simulink model "FOC_ctrl"  (R2025b)
settings: Solver=FixedStepAuto  StartTime=0.0  StopTime=Tstop  FixedStep=p.FastTs  RelTol=1e-3
undefined symbols (not defined in the file): angleDeg, c, Inverter, m, Motor, p, torqueNm, Tstop, we
libraries: simulink x5, fl_lib x4, nesl_utility x3, dspsigops x2, ee_lib x1
(part 1 of 3)
Description:
  | Release 2.0.11
settings Model: Creator=dehc5899  LastModifiedBy=dehc5899
settings SolverCC: AutoInsertRateTranBlk=on

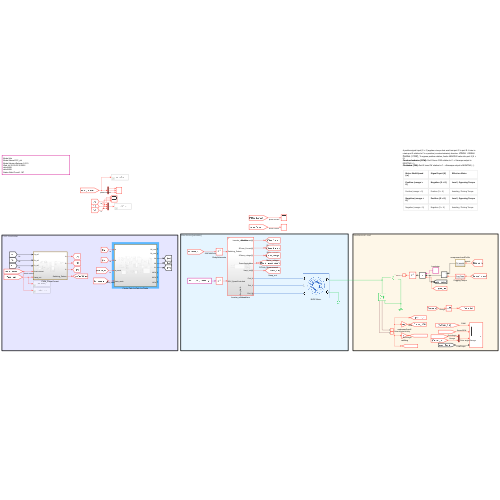
[thumbnail: Simulink's stored preview of the top-level diagram]
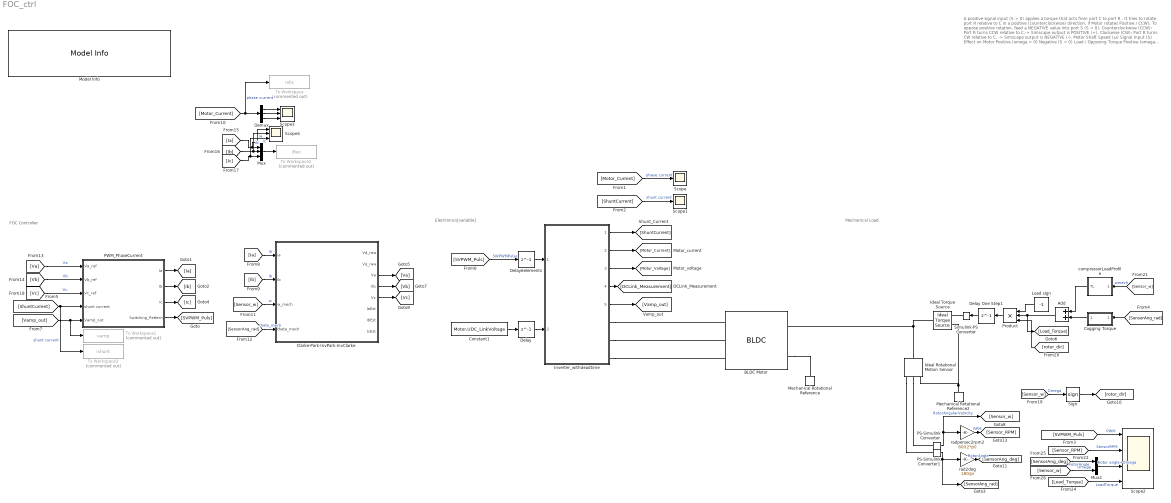
== system FOC_ctrl ==
  note: FOC Controller
  note: A positive signal input (S > 0) applies a torque that acts from port C to port R . It tries to rotate port R relative to C in a positive (counterclockwise) direction. if Motor rotates Positive / CCW), To oppose positive rotation, feed a NEGATIVE value into port S (S < 0).
      | Counterclockwise (CCW): Port R turns CCW relative to C.-> Simscape output is POSITIVE (+).
      | Clockwise (CW): Port R turns CW relative to C. -> Simscape output is NEGATIVE (-).
      |
      | Motor Shaft Speed (ω)
      | Signal Input (S)
      | Effect on Motor
      |
      | Positive (omega > 0)
      | Negative (S < 0)
      | Load / Opposing Torque
      |
      | Positive (omega > 0)
      | Positive (S > 0)
      | Assisting / Driving Torque
      |
      | Negative (omega < 0)
      | Positive (S > 0)
      | Load / Opposing Torque
      |
      | Negative (omega < 0)
      | Negative (S < 0)
      | Assisting / Driving Torque
  note: Electronics[variable]
  note: Mechanical Load
  Add : Sum
  BLDC Motor : ee_lib/Electromechanical/Permanent Magnet/BLDC  port_option=ee.enum.threePhasePort.expanded  rotor_param=ee.enum.pmsm.backemf.tabulatedbackemf  pm_flux_linkage=0.03 Wb  theta_constant=pi / 12 rad  emf_max=9.6 V  w_meas=Motor.bemfMeasSpeed rpm  DphiDtheta_tab=[0, -.1528, -.1528, .1528, .1528, 0] Wb/rad  back_emf_tab=BEMF_shape V  rotor_angle_tab=theta_mech deg  nPolePairs=Motor.PP_NumberOfPolePairs  axes_param=ee.enum.rotorangle.daxis  winding_type=ee.enum.electromech.statorconfiguration.wye  stator_param=ee.enum.statorparam.LsLmMs  machine_param=ee.enum.dqparameterization.constant  Ld=0.00022 H  Lq=0.00022 H  idVec=[-200, 0, 200] A  iqVec=[-200, 0, 200] A  LdMatrix=0.00022 * ones(3, 3) H  LqMatrix=0.00022 * ones(3, 3) H  L0=0.00016 H  Ls=Motor.Ls H  Lm=Motor.Lm H  Ms=Motor.Ms H  Rs=Motor.R_StatorResistance Ohm  zero_sequence=ee.enum.park.zerosequence.exclude  loss_param=ee.enum.ironloss.empirical  losses_oc=[0, 0, 0] W  losses_sc=[0, 0, 0] W  f_losses=60 Hz  Isc_losses=95 A  J=Motor.J_Inertia kg*m^2  lam=Motor.F_FrictionCoeff N*m*s/rad  i_d_specify=off  i_d_priority=None  i_d=0 A  i_d_nominal_specify=off  i_d_nominal_value=1  i_d_nominal_unit=A  i_q_specify=off  i_q_priority=None  i_q=0 A  i_q_nominal_specify=off  i_q_nominal_value=1  i_q_nominal_unit=A  torque_specify=off  torque_priority=None  torque=0 N*m  torque_nominal_specify=off  torque_nominal_value=1  torque_nominal_unit=N*m  angular_velocity_specify=on  angular_velocity_priority=Low  angular_velocity=Motor.wm0_InitialRotorSpeed rpm  angular_velocity_nominal_specify=off  angular_velocity_nominal_value=Motor.nNom_NominalSpeedrpm  angular_velocity_nominal_unit=rpm  angular_position_specify=on  angular_position_priority=Low  angular_position=Motor.thm0_InitialRotorAngle rad  angular_position_nominal_specify=off  angular_position_nominal_value=Motor.thm0_InitialRotorAngle  angular_position_nominal_unit=deg  alpha=3.93e-3 1/K  alpha_flux=-0.001 1/K  Tmeas=298.15 K  stator_thermal_mass=100 J/K  rotor_thermal_mass=200 J/K  Rm_percent_rotor=90  Rd_percent_rotor=30  temperatureA_specify=off  temperatureA_priority=High  temperatureA=25 degC  temperatureA_nominal_specify=off  temperatureA_nominal_value=1  temperatureA_nominal_unit=degC  temperatureB_specify=off  temperatureB_priority=High  temperatureB=25 degC  temperatureB_nominal_specify=off  temperatureB_nominal_value=1  temperatureB_nominal_unit=degC  temperatureC_specify=off  temperatureC_priority=High  temperatureC=25 degC  temperatureC_nominal_specify=off  temperatureC_nominal_value=1  temperatureC_nominal_unit=degC  temperatureR_specify=off  temperatureR_priority=High  temperatureR=25 degC  temperatureR_nominal_specify=off  temperatureR_nominal_value=1  temperatureR_nominal_unit=degC
      settings: InternalSimscapePortConfiguration="{\"Bottom\":[],\"Left\":[{\"id\":\"a\",\"label\":\"a\",\"type\":\"foundation.electrical.electrical\"},{\"id\":\"b\",\"label\":\"b\",\"type\":\"foundation.electrical.electrical\"},{\"id\":\"c\",\"label\":\"c\",\"type\":\"foundation.electrical.electrical\"}],\"Right\":[{\"id\":\"R\",\"label\":\"R\",\"type\":\"foundation.mechanical.rotational.rotational\"},{\"id\":\"C\",\"label\":\"C\",\"type\":\"foundation.mechanical.rotational.rotational\"}],\"Top\":[]}"
  Clarke-Park-InvPark-InvClarke : Subsystem
  Cogging Torque : Subsystem
      settings: PortSchema="{\"entries\":[{\"content\":{\"sides\":[{\"content\":{\"connectorIds\":[\"Out1\"]},\"type\":\"ConnectorPlacement.EquallySpacedRectSide\",\"uuid\":\"e72dd149-be6c-473d-b9a6-ab382dc36dd8\"},{\"content\":{\"connectorIds\":[\"In1\"],\"side\":\"RIGHT\"},\"type\":\"ConnectorPlacement.EquallySpacedRectSide\",\"uuid\":\"d6dbddf8-c929-46f7-8e18-d8605da261d8\"},{\"content\":{\"side\":\"TOP\"},\"type\":\"ConnectorPlacement.EquallySpacedRectSide\",\"uuid\":\"d97b9a66-7b14-44a9-8763-71570facd52d\"},{\"content\":{\"side\":\"BOTTOM\"},\"type\":\"ConnectorPlacement.EquallySpacedRectSide\",\"uuid\":\"30e90f76-fd4e-40c6-9e4e-ba219d693512\"}]},\"type\":\"ConnectorPlacement.EquallySpacedConnector\",\"uuid\":\"ce9d67e2-aed0-4e64-a6bd-15c2f7731a50\"}],\"packageUris\":[\"http://schema.mathworks.com/mf0/Connector/R2020b\"],\"version\":\"1.0\"}"
  Constant1 : Constant  Value=Motor.UDC_LinkVoltage
  Delay : Delay  DelayLength=1  InitialCondition=Inverter.UDC_LinkVoltage_Max  InputProcessing=Columns as channels (frame based)
  Delay One Step1 : Delay  DelayLength=1
  Delay6elements : Delay  DelayLength=1  InitialCondition=[0 0 0 0 0 0]
  Demux : Demux  Outputs=3
  Ideal Rotational Motion Sensor : fl_lib/Mechanical/Mechanical Sensors/Ideal Rotational Motion Sensor  reference=foundation.enum.MeasurementReference.difference  acceleration_port=false  velocity_port=true  position_port=true  wrap_angle=true  offset=Motor.thm0_InitialRotorAngle rad
  Ideal Torque Source : fl_lib/Mechanical/Mechanical Sources/Ideal Torque Source
  Inverter_withdeadtime : Subsystem  ReferencedSubsystem=inverter_withdtime
      settings: PortSchema="{\"entries\":[{\"content\":{\"sides\":[{\"content\":{\"connectorIds\":[\"In1\",\"In2\"]},\"type\":\"ConnectorPlacement.EquallySpacedRectSide\",\"uuid\":\"c4e4a499-a73b-47b6-b9d4-05a0b5c00da1\"},{\"content\":{\"connectorIds\":[\"Out1\",\"Out2\",\"Out3\",\"Out4\",\"Out5\",\"RConn1\",\"RConn2\",\"RConn3\"],\"side\":\"RIGHT\"},\"type\":\"ConnectorPlacement.EquallySpacedRectSide\",\"uuid\":\"f55443ed-1206-46a2-9a95-70ed1e950cf9\"},{\"content\":{\"side\":\"TOP\"},\"type\":\"ConnectorPlacement.EquallySpacedRectSide\",\"uuid\":\"cf76199e-050b-45cf-ab73-853bf2c84fa8\"},{\"content\":{\"connectorIds\":[\"RConn4\"],\"side\":\"BOTTOM\"},\"type\":\"ConnectorPlacement.EquallySpacedRectSide\",\"uuid\":\"91869a37-cdc1-4525-aadb-c80a51613b54\"}]},\"type\":\"ConnectorPlacement.EquallySpacedConnector\",\"uuid\":\"fb7c01bd-e96a-47ac-9a1b-b2a6f4f5bd80\"}],\"packageUris\":[\"http://schema.mathworks.com/mf0/Connector/R2020b\"],\"version\":\"1.0\"}"
  Load sign : Constant  Value=-1
  Mechanical Rotational Reference : fl_lib/Mechanical/Rotational Elements/Mechanical Rotational Reference
  Mechanical Rotational Reference2 : fl_lib/Mechanical/Rotational Elements/Mechanical Rotational Reference
  Model Info : simulink/Model-Wide Utilities/Model Info  Frame=on  DisplayStringWithTags=|  HorizontalTextAlignment=Left  LeftAlignmentValue=0.02
      | Model Info
      | Model Name:%<ModelName>
      | Model Version:%<Description>
      | %<Created>
      | %<Creator>
      | %<LastModifiedBy>
      | Native Build Count:%<ModelVersion>
  Mux : Mux  Inputs=3
  Mux2 : Mux  Inputs=2
  PS-Simulink Converter : nesl_utility/PS-Simulink Converter  PhysicalDomain=network_engine_domain  SubClassName=ps_output  LeftPortType=input  RightPortType=output  PseudoPeriodic=off  Frequencies=[]  VectorFormat=inherit  Unit=inherit  AffineConversion=off
  PS-Simulink Converter1 : nesl_utility/PS-Simulink Converter  PhysicalDomain=network_engine_domain  SubClassName=ps_output  LeftPortType=input  RightPortType=output  PseudoPeriodic=off  Frequencies=[]  VectorFormat=inherit  Unit=inherit  AffineConversion=off
  PWM_PhaseCurrent : Subsystem
  Product : Product  Inputs=3
  Scope : Scope
      settings: ActiveDisplayYMinimum=-20.416149345387971  ActiveDisplayYMaximum=25.22580313543488  DataLoggingVariableName=ScopeData4
  Scope1 : Scope
      settings: ActiveDisplayYMinimum=-6.3618713706725121  ActiveDisplayYMaximum=11.690256831370988  DataLoggingVariableName=ScopeData9
  Scope2 : Scope  NumInputPorts=4
      settings: ActiveDisplayYMinimum=-0.12499999999999997  ActiveDisplayYMaximum=1.125  DataLoggingVariableName=ScopeData5
  Scope3 : Scope  NumInputPorts=3
      settings: ActiveDisplayYMinimum=-12.058935324686422  ActiveDisplayYMaximum=12.950717402584473  DataLoggingVariableName=ScopeData23
  Scope4 : Scope  NumInputPorts=3
      settings: ActiveDisplayYMinimum=-2.083290326404279  ActiveDisplayYMaximum=1.1649120394540577  DataLoggingVariableName=ScopeData17
  Sign : Signum
  Simulink-PS Converter : nesl_utility/Simulink-PS Converter  PhysicalDomain=network_engine_domain  SubClassName=ps_input  LeftPortType=input  RightPortType=output  PseudoPeriodic=off  Frequencies=[]  NoiseDistribution=none  NoiseParameters=[]  Unit=1  AffineConversion=off  FilteringAndDerivatives=provide  SimscapeFilterOrder=1  InputFilterTimeConstant=0.001  UdotUserProvided=0
  To Workspace : ToWorkspace  Commented=on  VariableName=iabc  SaveFormat=Timeseries  SampleTime=-1
  To Workspace1 : ToWorkspace  Commented=on  VariableName=vamp  SaveFormat=Timeseries  SampleTime=-1
  To Workspace2 : ToWorkspace  Commented=on  VariableName=iRec  SaveFormat=Timeseries  SampleTime=-1
  To Workspace3 : ToWorkspace  Commented=on  VariableName=ishunt  SaveFormat=Timeseries  SampleTime=-1
  compressorLoadProfile : Subsystem
  rad2deg : Gain  Gain=180/pi
  radpersec2rpm2 : Gain  Gain=60/(2*pi)
  wires:
  PWM_PhaseCurrent/1(Ia) -> [Ia]
  PWM_PhaseCurrent/2(Ib) -> [Ib]
  Inverter_withdeadtime/4 -> [DCLink_Measurement]
  [SVPWM_Puls] -> Delay6elements/1  "SWPWMPulse"
  Inverter_withdeadtime/3 -> [Motor_Voltage]
  Inverter_withdeadtime/2 -> [Motor_Current]
  Inverter_withdeadtime/1 -> [ShuntCurrent]
  Delay/1 -> Inverter_withdeadtime/2
  Constant1/1 -> Delay/1
  Delay6elements/1 -> Inverter_withdeadtime/1
  PWM_PhaseCurrent/3(Ic) -> [Ic]
  [SensorAng_rad] -> Cogging Torque/1(Theta)
  PS-Simulink Converter/1 -> radpersec2rpm2/1, [Sensor_w]  "RotorAngularVelocity"
  rad2deg/1 -> [SensorAng_deg]  "RotorAngle"
  [Load_Torque] -> Scope2/4  "LoadTorque"
  PS-Simulink Converter1/1 -> [SensorAng_rad], rad2deg/1
  [Sensor_w] -> Mux2/2  "Omega"
  Cogging Torque/1(Tcog) -> Add/2
  Add/1 -> Product/2, [Load_Torque]
  [SensorAng_deg] -> Mux2/1  "RotorAngle"
  [SVPWM_Puls] -> Scope2/1  "PWM"
  radpersec2rpm2/1 -> [Sensor_RPM]  "RPM"
  Mux2/1 -> Scope2/3  "Rotor angle+Omega"
  [Sensor_RPM] -> Scope2/2  "SensorRPM"
  PWM_PhaseCurrent/4(Switching_Pattern) -> [SVPWM_Puls]
  [Motor_Current] -> Scope/1  "phase current"
  [ShuntCurrent] -> Scope1/1  "shunt current"
  [ShuntCurrent] -> PWM_PhaseCurrent/4(shunt current), To Workspace3/1  "shunt current"
  Inverter_withdeadtime/5 -> [Vamp_out]
  [Vamp_out] -> To Workspace1/1, PWM_PhaseCurrent/5(Vamp_out)
  [Ib] -> Scope4/2, Mux/2  "ib"
  [Ia] -> Scope4/1, Mux/1  "ia"
  [Ic] -> Scope4/3, Mux/3  "ic"
  [Ib] -> Clarke-Park-InvPark-InvClarke/2(ib)  "ib"
  [Ia] -> Clarke-Park-InvPark-InvClarke/1(ia)  "ia"
  [Motor_Current] -> To Workspace/1, Demux/1  "phase current"
  Demux/1 -> Scope3/1
  Demux/2 -> Scope3/2
  Demux/3 -> Scope3/3
  Mux/1 -> To Workspace2/1
  [Sensor_w] -> Clarke-Park-InvPark-InvClarke/3("w_mech ")  "w"
  [SensorAng_rad] -> Clarke-Park-InvPark-InvClarke/4("theta_mech ")  "theta_mech"
  Clarke-Park-InvPark-InvClarke/3(Va) -> [Va]
  Clarke-Park-InvPark-InvClarke/4(Vb) -> [Vb]
  Clarke-Park-InvPark-InvClarke/5(Vc) -> [Vc]
  [Vc] -> PWM_PhaseCurrent/3(Vc_ref)  "Vc"
  [Vb] -> PWM_PhaseCurrent/2(Vb_ref)  "Vb"
  [Va] -> PWM_PhaseCurrent/1(Va_ref)  "Va"
  Product/1 -> Delay One Step1/1
  [Sensor_w] -> Sign/1  "Omega"
  Sign/1 -> [rotor_dir]
  Load sign/1 -> Product/1
  [rotor_dir] -> Product/3
  Delay One Step1/1 -> Simulink-PS Converter/1
  [Sensor_w] -> compressorLoadProfile/1(wmech)  "wmech"
  compressorLoadProfile/1(TL) -> Add/1
  connections:
  BLDC Motor/RConn2 -- Mechanical Rotational Reference/LConn1
  Inverter_withdeadtime/RConn1 -- BLDC Motor/LConn1
  Inverter_withdeadtime/RConn2 -- BLDC Motor/LConn2
  Inverter_withdeadtime/RConn3 -- BLDC Motor/LConn3
  Mechanical Rotational Reference2/LConn1 -- Ideal Rotational Motion Sensor/RConn1 -- Ideal Torque Source/RConn2
  Ideal Torque Source/LConn1 -- Ideal Rotational Motion Sensor/LConn1 -- BLDC Motor/RConn1
  Ideal Rotational Motion Sensor/RConn3 -- PS-Simulink Converter1/LConn1
  Ideal Rotational Motion Sensor/RConn2 -- PS-Simulink Converter/LConn1
  Simulink-PS Converter/RConn1 -- Ideal Torque Source/RConn1

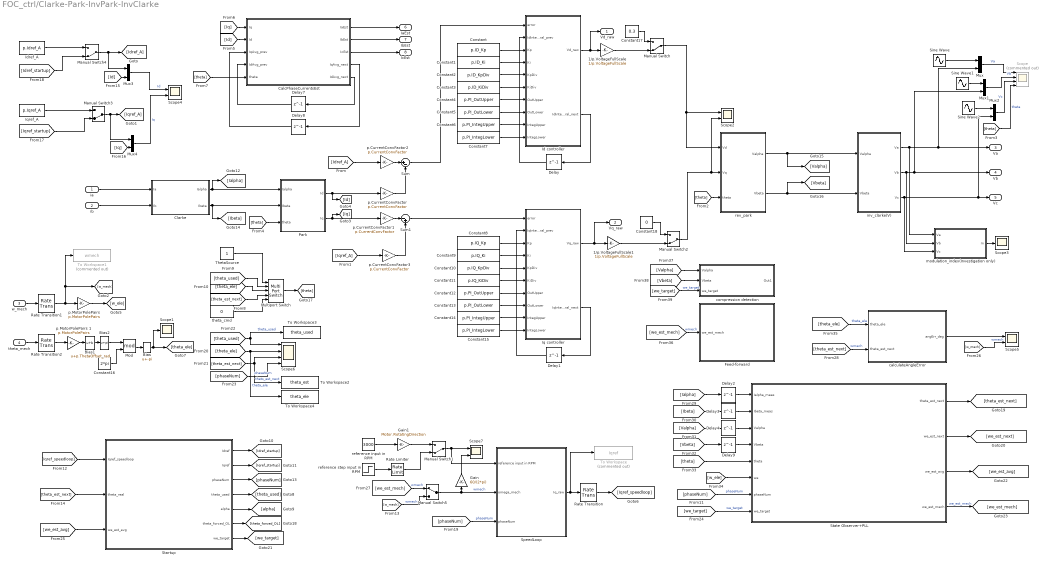
== system FOC_ctrl/Clarke-Park-InvPark-InvClarke ==
  ia : Inport
  ib : Inport  Port=2
  "w_mech " : Inport  Port=3
  "theta_mech " : Inport  Port=4
  1/p.VoltageFullScale : Gain  Gain=1/p.VoltageFullScale
  1/p.VoltageFullScale1 : Gain  Gain=1/p.VoltageFullScale
  Bias : Bias  Bias=-pi  SaturateOnIntegerOverflow=off
  Bias1 : Bias  Bias=p.ThetaOffset_rad  SaturateOnIntegerOverflow=off
  Bias2 : Bias  Bias=pi  SaturateOnIntegerOverflow=off
  CalcPhaseCurrentsEst : MATLAB Function  TreatAsAtomicUnit=on
  Clarke : MATLAB Function  TreatAsAtomicUnit=on
  Constant : Constant  Value=p.ID_Kp
  Constant1 : Constant  Value=p.ID_Ki
  Constant10 : Constant  Value=p.IQ_KpDiv
  Constant11 : Constant  Value=p.IQ_KiDiv
  Constant12 : Constant  Value=p.PI_OutUpper
  Constant13 : Constant  Value=p.PI_OutLower
  Constant14 : Constant  Value=p.PI_IntegUpper
  Constant15 : Constant  Value=p.PI_IntegLower
  Constant16 : Constant  Value=2*pi
  Constant17 : Constant  Value=0.3
  Constant18 : Constant  Value=0
  Constant2 : Constant  Value=p.ID_KpDiv
  Constant3 : Constant  Value=p.ID_KiDiv
  Constant4 : Constant  Value=p.PI_OutUpper
  Constant5 : Constant  Value=p.PI_OutLower
  Constant6 : Constant  Value=p.PI_IntegUpper
  Constant7 : Constant  Value=p.PI_IntegLower
  Constant8 : Constant  Value=p.IQ_Kp
  Constant9 : Constant  Value=p.IQ_Ki
  Delay{,1..4,7..9} (8 alike) : Delay  DelayLength=1  SampleTime=p.Ts
  Feed-forward : Subsystem
  Gain : Gain  Gain=60/(2*pi)
  Gain1 : Gain  Gain=Motor.RotatingDirection
  Id controller : MATLAB Function  TreatAsAtomicUnit=on
  Idref_A : Constant  Value=p.Idref_A
  Iq controller : MATLAB Function  TreatAsAtomicUnit=on
  Iqref_A : Constant  Value=p.Iqref_A
  Manual Switch{,1..4} (5 alike) : ManualSwitch  CurrentSetting=0
  Manual Switch5 : ManualSwitch
  Mod : Math  Operator=mod
  Multiport Switch : MultiPortSwitch  Inputs=4  SaturateOnIntegerOverflow=off  InputSameDT=off
  Mux{,1..4} (5 alike) : Mux  Inputs=2
  Park : MATLAB Function  TreatAsAtomicUnit=on
  Rate Limiter : RateLimiter  RisingSlewLimit=1000  FallingSlewLimit=-1000  SampleTimeMode=inherited
  Rate Transition : RateTransition  OutPortSampleTime=p.Ts
  Rate Transition1 : RateTransition  OutPortSampleTime=p.Ts
  Rate Transition2 : RateTransition  OutPortSampleTime=p.Ts
  Scope : Scope  Commented=on  NumInputPorts=4
      settings: ActiveDisplayYMinimum=-1.2422809671746262  ActiveDisplayYMaximum=1.2510473620175615  DataLoggingVariableName=ScopeData28
  Scope1 : Scope
      settings: ActiveDisplayYMinimum=-3.9122097003518697  ActiveDisplayYMaximum=3.9252709994043578  DataLoggingVariableName=ScopeData29
  Scope{2,4..5,7} (4 alike) : Scope  NumInputPorts=2
      Scope2 settings: ActiveDisplayYMinimum=-1.25  ActiveDisplayYMaximum=1.25  DataLoggingVariableName=ScopeData24
      Scope4 settings: ActiveDisplayYMinimum=-20.880653468228683  ActiveDisplayYMaximum=14.701115824739801  DataLoggingVariableName=ScopeData30
      Scope5 settings: ActiveDisplayYMinimum=-117.96274425061029  ActiveDisplayYMaximum=161.83782725060485  DataLoggingVariableName=ScopeData39
      Scope7 settings: ActiveDisplayYMinimum=2312.5  ActiveDisplayYMaximum=4187.5  DataLoggingVariableName=ScopeData27
  Scope3 : Scope
      settings: ActiveDisplayYMinimum=-0.14724423081589327  ActiveDisplayYMaximum=1.4824902174457719  DataLoggingVariableName=ScopeData25
  Scope6 : Scope  NumInputPorts=4
      settings: ActiveDisplayYMinimum=-3.9259634965545649  ActiveDisplayYMaximum=3.9265413925231916  DataLoggingVariableName=ScopeData35
  Sine Wave : Sin  Amplitude=m  Frequency=we  SampleTime=p.Ts
  Sine Wave1 : Sin  Amplitude=m  Frequency=we  Phase=-2*pi/3  SampleTime=p.Ts
  Sine Wave2 : Sin  Amplitude=m  Frequency=we  Phase=2*pi/3  SampleTime=p.Ts
  SpeedLoop : Subsystem  TreatAsAtomicUnit=on  SystemSampleTime=p.SpeedTs
  Startup : Subsystem
  State Observer+PLL : Subsystem
  Sum : Sum  Inputs=|+-
  Sum1 : Sum  Inputs=|-+
  ThetaSource : Constant
  To Workspace : ToWorkspace  Commented=on  VariableName=Iqref  SaveFormat=Timeseries  SampleTime=-1
  To Workspace1 : ToWorkspace  Commented=on  VariableName=wmech  SaveFormat=Timeseries  SampleTime=-1
  To Workspace2 : ToWorkspace  VariableName=theta_est  SaveFormat=Timeseries  SampleTime=-1
  To Workspace3 : ToWorkspace  VariableName=theta_used  SaveFormat=Timeseries  SampleTime=-1
  To Workspace4 : ToWorkspace  VariableName=theta_ele  SaveFormat=Timeseries  SampleTime=-1
  calculateAngleError : MATLAB Function  TreatAsAtomicUnit=on
  compression detection : Subsystem
  inv_clarke(V) : MATLAB Function  TreatAsAtomicUnit=on
  modulation_index(Investigation only) : MATLAB Function  TreatAsAtomicUnit=on
  p.CurrentConvFactor{,1..3} (4 alike) : Gain  Gain=p.CurrentConvFactor
  "p.MotorPolePairs " : Gain  Gain=p.MotorPolePairs
  p.MotorPolePairs 1 : Gain  Gain=p.MotorPolePairs
  reference input in RPM : Constant  Value=3000
  reference step input in RPM : Step  Before=2500  After=4000  SampleTime=0
  rev_park : MATLAB Function  TreatAsAtomicUnit=on
  theta_cmd : Constant  Value=0
  Vd_raw : Outport
  Vq_raw : Outport  Port=2
  Va : Outport  Port=3
  Vb : Outport  Port=4
  Vc : Outport  Port=5
  IaEst : Outport  Port=6
  IbEst : Outport  Port=7
  IcEst : Outport  Port=8
  wires:
  p.CurrentConvFactor/1 -> Sum/2
  Sum1/1 -> Iq controller/1(error)
  Constant3/1 -> Id controller/6(KiDiv)
  [Idref_A] -> p.CurrentConvFactor2/1
  Constant8/1 -> Iq controller/3(Kp)
  Constant2/1 -> Id controller/5(KpDiv)
  Iq controller/2(IqIntegral_next) -> Delay1/1
  ia/1 -> Clarke/1(Ia)
  Id controller/2(IdIntegral_next) -> Delay/1
  p.CurrentConvFactor2/1 -> Sum/1
  Park/2(Iq) -> [Iq], p.CurrentConvFactor1/1
  Park/1(Id) -> [Id], p.CurrentConvFactor/1
  ib/1 -> Clarke/2(Ib)
  p.CurrentConvFactor3/1 -> Sum1/2
  p.CurrentConvFactor1/1 -> Sum1/1
  Constant/1 -> Id controller/3(Kp)
  Iq controller/1(Vq_raw) -> Vq_raw/1, 1/p.VoltageFullScale1/1
  [Iqref_A] -> p.CurrentConvFactor3/1
  Clarke/1(Ialpha) -> Park/1(Ialpha), [Ialpha]
  Clarke/2(Ibeta) -> Park/2(Ibeta), [Ibeta]
  Constant9/1 -> Iq controller/4(Ki)
  Constant7/1 -> Id controller/10(IntegLower)
  Constant10/1 -> Iq controller/5(KpDiv)
  Iqref_A/1 -> Manual Switch3/1
  Manual Switch4/1 -> Mux3/1, [Idref_A]
  Sum/1 -> Id controller/1(error)
  Id controller/1(Vd_raw) -> 1/p.VoltageFullScale/1, Vd_raw/1
  Constant12/1 -> Iq controller/7(OutUpper)
  Constant1/1 -> Id controller/4(Ki)
  Constant6/1 -> Id controller/9(IntegUpper)
  Constant5/1 -> Id controller/8(OutLower)
  Delay/1 -> Id controller/2(IdIntegral_prev)
  Delay1/1 -> Iq controller/2(IqIntegral_prev)
  Constant11/1 -> Iq controller/6(KiDiv)
  Constant15/1 -> Iq controller/10(IntegLower)
  Constant14/1 -> Iq controller/9(IntegUpper)
  Constant13/1 -> Iq controller/8(OutLower)
  Constant4/1 -> Id controller/7(OutUpper)
  inv_clarke(V)/1(Va) -> Mux/2, Va/1, modulation_index(Investigation only)/1(Va)
  modulation_index(Investigation only)/1(m) -> Scope3/1
  inv_clarke(V)/2(Vb) -> modulation_index(Investigation only)/2(Vb), Mux1/2, Vb/1
  Manual Switch2/1 -> Scope2/2, rev_park/2(Vq)
  Manual Switch/1 -> rev_park/1(Vd), Scope2/1
  [theta] -> Scope/4  "theta"
  inv_clarke(V)/3(Vc) -> modulation_index(Investigation only)/3(Vc), Mux2/2, Vc/1
  [theta] -> rev_park/3(theta)
  [theta] -> Park/3(theta)
  reference input in RPM/1 -> Gain1/1
  Manual Switch1/1 -> SpeedLoop/1(reference input in RPM), Scope7/1
  reference step input in RPM/1 -> Rate Limiter/1
  Manual Switch5/1 -> SpeedLoop/2(omega_mech), Gain/1  "wmech"
  Rate Transition/1 -> [Iqref_speedloop]
  Gain/1 -> Scope7/2
  SpeedLoop/1(Iq_raw) -> To Workspace/1, Rate Transition/1
  CalcPhaseCurrentsEst/5(IdAvg_next) -> Delay7/1
  CalcPhaseCurrentsEst/2(IbEst) -> IbEst/1
  CalcPhaseCurrentsEst/3(IcEst) -> IcEst/1
  CalcPhaseCurrentsEst/1(IaEst) -> IaEst/1
  Delay8/1 -> CalcPhaseCurrentsEst/3(IqAvg_prev)
  CalcPhaseCurrentsEst/4(IqAvg_next) -> Delay8/1
  [Id] -> CalcPhaseCurrentsEst/2(Id)
  [theta] -> CalcPhaseCurrentsEst/5(theta)
  Delay7/1 -> CalcPhaseCurrentsEst/4(IdAvg_prev)
  [Iq] -> CalcPhaseCurrentsEst/1(Iq)
  [Ialpha] -> Delay2/1
  [Ibeta] -> Delay3/1
  [w_ele] -> State Observer+PLL/6(we)
  [Vbeta] -> Delay9/1
  [Valpha] -> Delay4/1
  State Observer+PLL/1(theta_est_next) -> [theta_est_next]
  State Observer+PLL/2(we_est_next) -> [we_est_next]
  [theta] -> State Observer+PLL/5(theta)
  rev_park/1(Valpha) -> [Valpha], inv_clarke(V)/1(Valpha)
  rev_park/2(Vbeta) -> [Vbeta], inv_clarke(V)/2(Vbeta)
  Delay2/1 -> State Observer+PLL/1(Ialpha_meas)
  Delay3/1 -> State Observer+PLL/2(Ibeta_meas)
  Delay4/1 -> State Observer+PLL/3(Valpha)
  Delay9/1 -> State Observer+PLL/4(Vbeta)
  "w_mech "/1 -> Rate Transition1/1
  "p.MotorPolePairs "/1 -> [w_ele]
  Startup/1(Idref) -> [Idref_startup]
  Startup/2(Iqref) -> [Iqref_startup]
  Startup/4(theta_used) -> [theta_used]
  Startup/3(phaseNum) -> [phaseNum]
  Startup/5(alpha) -> [alpha]
  "theta_mech "/1 -> Rate Transition2/1
  p.MotorPolePairs 1/1 -> Bias1/1
  Constant16/1 -> Mod/2
  ThetaSource/1 -> Multiport Switch/1
  Multiport Switch/1 -> [theta]
  [theta_est_next] -> Multiport Switch/4
  Mod/1 -> Bias/1
  Startup/6(theta_forced_OL) -> [theta_forced_OL]
  [theta_used] -> Multiport Switch/2
  Bias/1 -> [theta_ele], Scope1/1
  [theta_ele] -> Multiport Switch/3
  1/p.VoltageFullScale/1 -> Manual Switch/2
  Constant17/1 -> Manual Switch/1
  1/p.VoltageFullScale1/1 -> Manual Switch2/2
  Constant18/1 -> Manual Switch2/1
  Sine Wave/1 -> Mux/1
  Sine Wave1/1 -> Mux1/1
  Sine Wave2/1 -> Mux2/1
  Bias1/1 -> Bias2/1
  Mux/1 -> Scope/1  "Va"
  Mux1/1 -> Scope/2  "Vb"
  Mux2/1 -> Scope/3  "Vc"
  Rate Transition1/1 -> To Workspace1/1, [w_mech], "p.MotorPolePairs "/1
  Rate Transition2/1 -> p.MotorPolePairs 1/1
  [Iqref_speedloop] -> Startup/1("Iqref_speedloop ")
  [theta_est_next] -> Startup/2("theta_real ")
  theta_cmd/1 -> Multiport Switch/5
  Bias2/1 -> Mod/1
  Mux3/1 -> Scope4/1  "Id"
  Mux4/1 -> Scope4/2  "Iq"
  [Iq] -> Mux4/2
  [Id] -> Mux3/2
  [Iqref_startup] -> Manual Switch3/2
  Manual Switch3/1 -> Mux4/1, [Iqref_A]
  Gain1/1 -> Manual Switch1/1
  Idref_A/1 -> Manual Switch4/1
  [Idref_startup] -> Manual Switch4/2
  [phaseNum] -> SpeedLoop/3(phaseNum)  "phaseNum"
  [theta_used] -> Scope6/1, To Workspace3/1  "theta_used"
  [theta_ele] -> To Workspace4/1, Scope6/2  "theta_ele"
  [theta_est_next] -> To Workspace2/1, Scope6/3  "thets_est_next"
  [phaseNum] -> Scope6/4  "phaseNum"
  Rate Limiter/1 -> Manual Switch1/2
  [phaseNum] -> State Observer+PLL/7(phaseNum)  "phaseNum"
  Startup/7(we_target) -> [we_target]
  [we_target] -> State Observer+PLL/8(we_target)  "we_target"
  [we_est_avg] -> Startup/3(we_est_avg)
  State Observer+PLL/3(we_est_avg) -> [we_est_avg]
  [w_mech] -> Scope5/2  "wmech"
  State Observer+PLL/4(we_est_mech) -> [we_est_mech]  "we_est_mech"
  [w_mech] -> Manual Switch5/2  "wmech"
  [we_est_mech] -> Manual Switch5/1  "wmech"
  [theta_est_next] -> calculateAngleError/2(theta_est_next)  "wmech"
  [theta_ele] -> calculateAngleError/1(theta_ele)  "theta_ele"
  calculateAngleError/1(angErr_deg) -> Scope5/1
  [we_est_mech] -> Feed-forward/1(we_est_mech)  "wmech"
  [we_target] -> compression detection/3(we_target)  "we_target"
  [Vbeta] -> compression detection/2(Vbeta)
  [Valpha] -> compression detection/1(Valpha)

== system FOC_ctrl/Cogging Torque ==
  Theta : Inport
  Memory : Memory
  Scope3 : Scope
      settings: ActiveDisplayYMinimum=-0.048749999766971877  ActiveDisplayYMaximum=0.048749999963062271  DataLoggingVariableName=ScopeData6
  Variant Subsystem : Subsystem  Variant=on  EmptyChoice=on
  Tcog : Outport
  wires:
  Theta/1 -> Memory/1
  Variant Subsystem/1(Tcog) -> Scope3/1, Tcog/1
  Memory/1 -> Variant Subsystem/1(theta)

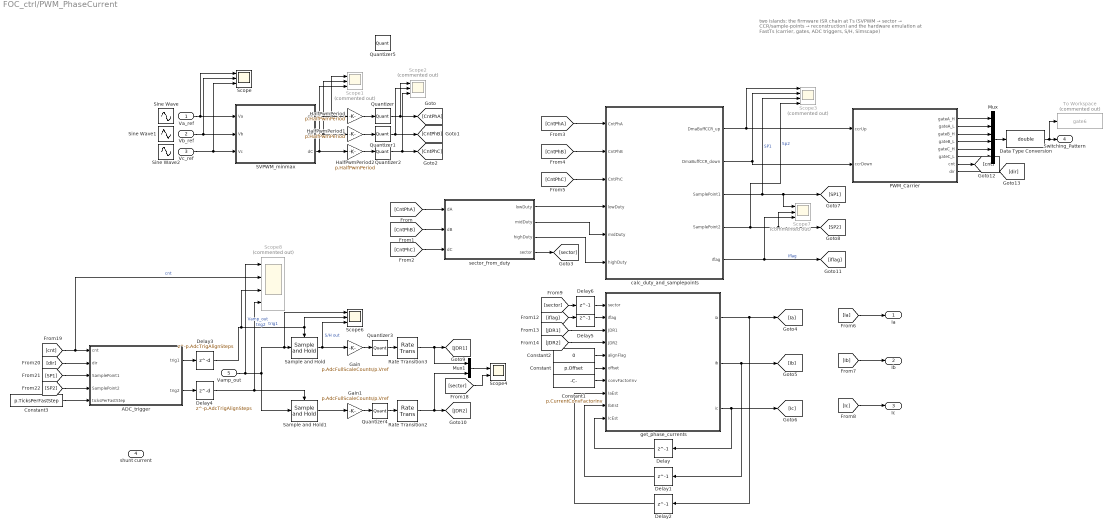
== system FOC_ctrl/PWM_PhaseCurrent ==
  note: two islands: the firmware ISR chain at Ts (SVPWM → sector → CCR/sample-points → reconstruction) and the hardware emulation at FastTs (carrier, gates, ADC triggers, S/H, Simscape)
  Va_ref : Inport
  Vb_ref : Inport  Port=2
  Vc_ref : Inport  Port=3
  shunt current : Inport  Port=4
  Vamp_out : Inport  Port=5
  ADC_trigger : MATLAB Function  TreatAsAtomicUnit=on
  Constant : Constant  Value=p.Offset
  Constant1 : Constant  Value=p.CurrentConvFactorInv
  Constant2 : Constant  Value=0
  Constant3 : Constant  Value=p.TicksPerFastStep
  Data Type Conversion : DataTypeConversion  OutDataTypeStr=double  SaturateOnIntegerOverflow=off  RndMeth=Floor
  Delay{,1..2,5} (4 alike) : Delay  DelayLength=1
  Delay3 : Delay  DelayLength=p.AdcTrigAlignSteps  InitialCondition=0  SampleTime=p.FastTs
  Delay4 : Delay  DelayLength=p.AdcTrigAlignSteps  InitialCondition=0  SampleTime=p.FastTs
  Delay6 : Delay  DelayLength=1  InitialCondition=1
  Gain : Gain  Gain=p.AdcFullScaleCounts/p.Vref
  Gain1 : Gain  Gain=p.AdcFullScaleCounts/p.Vref
  HalfPwmPeriod : Gain  Gain=p.HalfPwmPeriod
  HalfPwmPeriod1 : Gain  Gain=p.HalfPwmPeriod
  HalfPwmPeriod2 : Gain  Gain=p.HalfPwmPeriod
  Mux : Mux  Inputs=6
  Mux1 : Mux  Inputs=2
  PWM_Carrier : Subsystem  TreatAsAtomicUnit=on  SystemSampleTime=p.FastTs
  Quantizer{,1..2,5} (4 alike) : Quantizer  QuantizationInterval=p.TicksPerFastStep
  Quantizer3 : Quantizer  QuantizationInterval=1
  Quantizer4 : Quantizer  QuantizationInterval=1
  Rate Transition2 : RateTransition  OutPortSampleTime=p.Ts
  Rate Transition3 : RateTransition  OutPortSampleTime=p.Ts
  SVPWM_minmax : MATLAB Function  TreatAsAtomicUnit=on
  Sample and Hold : dspsigops/Sample and Hold  trig=Rising edge  initCond=0  latchinput=off
  Sample and Hold1 : dspsigops/Sample and Hold  trig=Rising edge  initCond=0  latchinput=off
  Scope : Scope  NumInputPorts=3
      settings: ActiveDisplayYMinimum=-1.7670802058532755  ActiveDisplayYMaximum=1.7615871298568744
  Scope1 : Scope  Commented=on  NumInputPorts=3
      settings: ActiveDisplayYMinimum=0.36044361461932012  ActiveDisplayYMaximum=0.40645121419536845
  Scope2 : Scope  Commented=on  NumInputPorts=3
      settings: ActiveDisplayYMinimum=1487.5  ActiveDisplayYMaximum=5312.5  DataLoggingVariableName=ScopeData2
  Scope3 : Scope  Commented=on  NumInputPorts=4
      settings: ActiveDisplayYMinimum=7.5000000000000036  ActiveDisplayYMaximum=152.5  DataLoggingVariableName=ScopeData7
  Scope4 : Scope  NumInputPorts=2
      settings: ActiveDisplayYMinimum=-4999.6249999999991  ActiveDisplayYMaximum=44996.625  DataLoggingVariableName=ScopeData15
  Scope6 : Scope  NumInputPorts=3
      settings: ActiveDisplayYMinimum=1.8375957763508237  ActiveDisplayYMaximum=1.98171120302503  DataLoggingVariableName=ScopeData19
  Scope7 : Scope  Commented=on  NumInputPorts=3
      settings: ActiveDisplayYMinimum=669.00000000000011  ActiveDisplayYMaximum=6049  DataLoggingVariableName=ScopeData20
  Scope8 : Scope  Commented=on  NumInputPorts=4
      settings: ActiveDisplayYMinimum=1.4717988133543585  ActiveDisplayYMaximum=3.2581616716597681  DataLoggingVariableName=ScopeData22
  Sine Wave : Sin  Amplitude=m  Frequency=we  SampleTime=p.Ts
  Sine Wave1 : Sin  Amplitude=m  Frequency=we  Phase=-2*pi/3  SampleTime=p.Ts
  Sine Wave2 : Sin  Amplitude=m  Frequency=we  Phase=2*pi/3  SampleTime=p.Ts
  To Workspace : ToWorkspace  Commented=on  VariableName=gate6  SaveFormat=Timeseries  SampleTime=-1
  calc_duty_and_samplepoints : MATLAB Function  TreatAsAtomicUnit=on
  get_phase_currents : MATLAB Function  TreatAsAtomicUnit=on
  sector_from_duty : MATLAB Function  TreatAsAtomicUnit=on
  Ia : Outport
  Ib : Outport  Port=2
  Ic : Outport  Port=3
  Switching_Pattern : Outport  Port=4
  wires:
  SVPWM_minmax/1(dA) -> HalfPwmPeriod/1, Scope1/1
  SVPWM_minmax/3(dC) -> HalfPwmPeriod2/1, Scope1/3
  SVPWM_minmax/2(dB) -> HalfPwmPeriod1/1, Scope1/2
  Va_ref/1 -> Scope/1, SVPWM_minmax/1(Va)
  Vb_ref/1 -> Scope/2, SVPWM_minmax/2(Vb)
  Vc_ref/1 -> Scope/3, SVPWM_minmax/3(Vc)
  HalfPwmPeriod1/1 -> Quantizer1/1
  HalfPwmPeriod/1 -> Quantizer/1
  HalfPwmPeriod2/1 -> Quantizer2/1
  Quantizer1/1 -> [CntPhB], Scope2/2
  Quantizer2/1 -> [CntPhC], Scope2/3
  Quantizer/1 -> [CntPhA], Scope2/1
  [CntPhA] -> sector_from_duty/1(dA)
  [CntPhB] -> sector_from_duty/2(dB)
  [CntPhC] -> sector_from_duty/3(dC)
  sector_from_duty/3(highDuty) -> calc_duty_and_samplepoints/6(highDuty)
  sector_from_duty/2(midDuty) -> calc_duty_and_samplepoints/5(midDuty)
  sector_from_duty/1(lowDuty) -> calc_duty_and_samplepoints/4(lowDuty)
  [CntPhA] -> calc_duty_and_samplepoints/1(CntPhA)
  [CntPhB] -> calc_duty_and_samplepoints/2(CntPhB)
  [CntPhC] -> calc_duty_and_samplepoints/3(CntPhC)
  sector_from_duty/4(sector) -> [sector]
  get_phase_currents/3(ic) -> [Ic], Delay/1
  Delay/1 -> get_phase_currents/10(IcEst)
  get_phase_currents/2(ib) -> [Ib], Delay1/1
  Delay1/1 -> get_phase_currents/9(IbEst)
  get_phase_currents/1(ia) -> [Ia], Delay2/1
  Delay2/1 -> get_phase_currents/8(IaEst)
  [Ia] -> Ia/1
  [Ib] -> Ib/1
  [Ic] -> Ic/1
  calc_duty_and_samplepoints/2(DmaBuffCCR_down) -> PWM_Carrier/2(ccrDown), Scope3/2
  calc_duty_and_samplepoints/1(DmaBuffCCR_up) -> PWM_Carrier/1(ccrUp), Scope3/1
  PWM_Carrier/1(gateA_H) -> Mux/1
  PWM_Carrier/2(gateA_L) -> Mux/2
  PWM_Carrier/3(gateB_H) -> Mux/3
  PWM_Carrier/4(gateB_L) -> Mux/4
  PWM_Carrier/5(gateC_H) -> Mux/5
  PWM_Carrier/6(gateC_L) -> Mux/6
  Mux/1 -> Data Type Conversion/1
  Data Type Conversion/1 -> To Workspace/1, Switching_Pattern/1
  Vamp_out/1 -> Scope8/1, Sample and Hold1/1, Scope6/1, Sample and Hold/1  "Vamp_out"
  Delay3/1 -> Scope8/3, Sample and Hold/Trigger, Scope6/2  "trig1"
  Delay4/1 -> Scope8/4, Sample and Hold1/Trigger  "trig2"
  Sample and Hold/1 -> Scope6/3, Gain/1  "S/H out"
  Sample and Hold1/1 -> Gain1/1
  Gain/1 -> Quantizer3/1
  Gain1/1 -> Quantizer4/1
  Quantizer3/1 -> Rate Transition3/1
  Quantizer4/1 -> Rate Transition2/1
  calc_duty_and_samplepoints/3(SamplePoint1) -> [SP1], Scope7/1, Scope3/3  "SP1"
  calc_duty_and_samplepoints/4(SamplePoint2) -> [SP2], Scope7/2, Scope3/4  "Sp2"
  [JDR2] -> get_phase_currents/4(JDR2)
  [JDR1] -> get_phase_currents/3(JDR1)
  calc_duty_and_samplepoints/5(iflag) -> Scope7/3, [iflag]  "Iflag"
  Constant/1 -> get_phase_currents/6(offset)
  Constant1/1 -> get_phase_currents/7(convFactorInv)
  Constant2/1 -> get_phase_currents/5(alignFlag)
  Mux1/1 -> Scope4/1
  [sector] -> Scope4/2
  PWM_Carrier/7(cnt) -> [cnt]
  PWM_Carrier/8(dir) -> [dir]
  [cnt] -> Scope8/2, ADC_trigger/1(cnt)  "cnt"
  [dir] -> ADC_trigger/2(dir)
  [SP1] -> ADC_trigger/3(SamplePoint1)
  [SP2] -> ADC_trigger/4(SamplePoint2)
  Constant3/1 -> ADC_trigger/5(ticksPerFastStep)
  ADC_trigger/1(trig1) -> Delay3/1
  ADC_trigger/2(trig2) -> Delay4/1
  Rate Transition3/1 -> [JDR1], Mux1/1
  Rate Transition2/1 -> [JDR2], Mux1/2
  [sector] -> Delay6/1
  Delay6/1 -> get_phase_currents/1(sector)
  [iflag] -> Delay5/1
  Delay5/1 -> get_phase_currents/2(iflag)

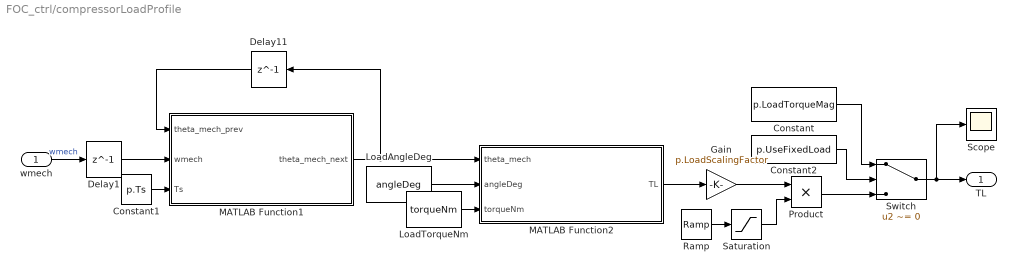
== system FOC_ctrl/compressorLoadProfile ==
  wmech : Inport
  Constant : Constant  Value=p.LoadTorqueMag
  Constant1 : Constant  Value=p.Ts
  Constant2 : Constant  Value=p.UseFixedLoad
  Delay1 : Delay  DelayLength=1  SampleTime=p.Ts
  Delay11 : Delay  DelayLength=1  SampleTime=p.Ts
  Gain : Gain  Gain=p.LoadScalingFactor
  LoadAngleDeg : Constant  Value=angleDeg
  LoadTorqueNm : Constant  Value=torqueNm
  MATLAB Function1 : MATLAB Function  TreatAsAtomicUnit=on
  MATLAB Function2 : MATLAB Function  TreatAsAtomicUnit=on
  Product : Product
  Ramp : simulink/Sources/Ramp  slope=p.loadRampSlope  start=p.Startup_T(1)  InitialOutput=0
  Saturation : Saturate  UpperLimit=1  LowerLimit=0
  Scope : Scope
      settings: ActiveDisplayYMinimum=-1  ActiveDisplayYMaximum=1  DataLoggingVariableName=ScopeData41
  Switch : Switch  Criteria=u2 ~= 0  SaturateOnIntegerOverflow=off  InputSameDT=off
  TL : Outport
  wires:
  Constant1/1 -> MATLAB Function1/3(Ts)
  LoadAngleDeg/1 -> MATLAB Function2/2(angleDeg)
  LoadTorqueNm/1 -> MATLAB Function2/3(torqueNm)
  wmech/1 -> Delay1/1  "wmech"
  MATLAB Function1/1(theta_mech_next) -> MATLAB Function2/1(theta_mech), Delay11/1
  Delay11/1 -> MATLAB Function1/1(theta_mech_prev)
  MATLAB Function2/1(TL) -> Gain/1
  Delay1/1 -> MATLAB Function1/2(wmech)
  Ramp/1 -> Saturation/1
  Saturation/1 -> Product/2
  Constant2/1 -> Switch/2
  Product/1 -> Switch/3
  Constant/1 -> Switch/1
  Switch/1 -> Scope/1, TL/1
  Gain/1 -> Product/1

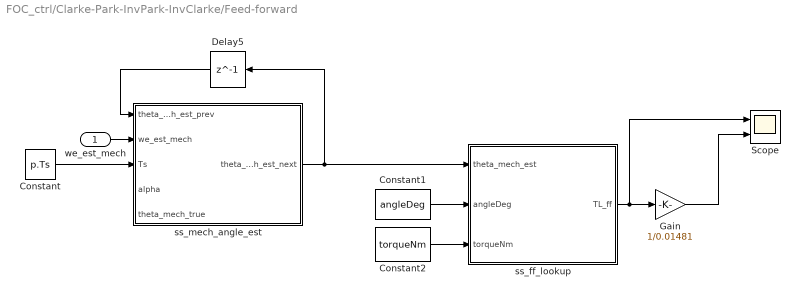
== system FOC_ctrl/Clarke-Park-InvPark-InvClarke/Feed-forward ==
  we_est_mech : Inport
  Constant : Constant  Value=p.Ts
  Constant1 : Constant  Value=angleDeg
  Constant2 : Constant  Value=torqueNm
  Delay5 : Delay  DelayLength=1  SampleTime=p.Ts
  Gain : Gain  Gain=1/0.01481
  Scope : Scope  NumInputPorts=2
      settings: ActiveDisplayYMinimum=-0.25620112617428942  ActiveDisplayYMaximum=0.73632857128938534  DataLoggingVariableName=ScopeData40
  ss_ff_lookup : MATLAB Function  TreatAsAtomicUnit=on
  ss_mech_angle_est : MATLAB Function  TreatAsAtomicUnit=on
  wires:
  ss_mech_angle_est/1(theta_mech_est_next) -> ss_ff_lookup/1(theta_mech_est), Delay5/1
  Delay5/1 -> ss_mech_angle_est/1(theta_mech_est_prev)
  Constant/1 -> ss_mech_angle_est/3(Ts)
  we_est_mech/1 -> ss_mech_angle_est/2(we_est_mech)
  Constant1/1 -> ss_ff_lookup/2(angleDeg)
  Constant2/1 -> ss_ff_lookup/3(torqueNm)
  ss_ff_lookup/1(TL_ff) -> Scope/1, Gain/1
  Gain/1 -> Scope/2

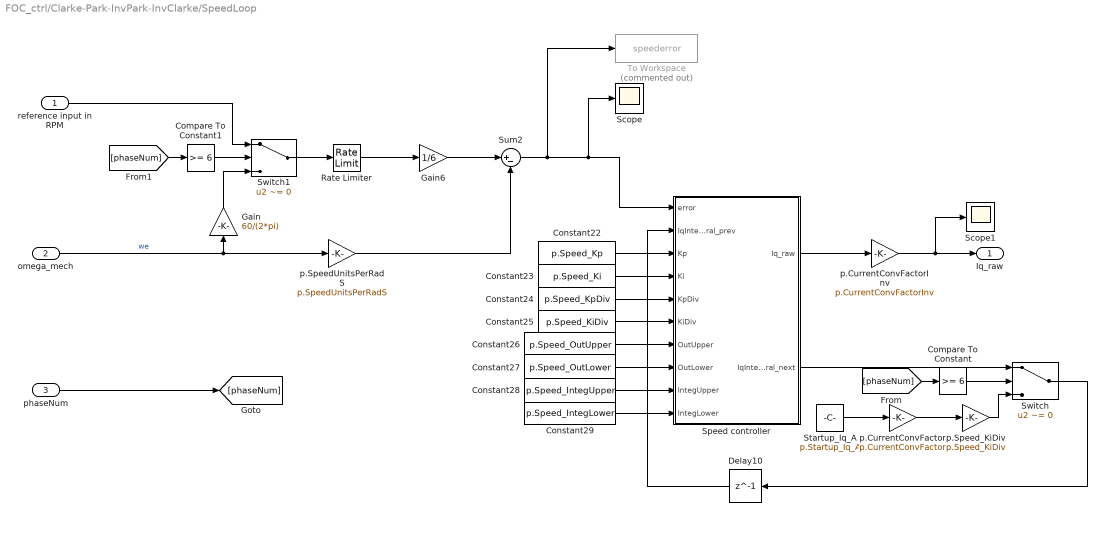
== system FOC_ctrl/Clarke-Park-InvPark-InvClarke/SpeedLoop ==
  reference input in RPM : Inport
  omega_mech : Inport  Port=2
  phaseNum : Inport  Port=3
  Compare To Constant : simulink/Logic and Bit Operations/Compare To Constant  relop=>=  const=6  OutDataTypeStr=boolean
  Compare To Constant1 : simulink/Logic and Bit Operations/Compare To Constant  relop=>=  const=6  OutDataTypeStr=boolean
  Constant22 : Constant  Value=p.Speed_Kp
  Constant23 : Constant  Value=p.Speed_Ki
  Constant24 : Constant  Value=p.Speed_KpDiv
  Constant25 : Constant  Value=p.Speed_KiDiv
  Constant26 : Constant  Value=p.Speed_OutUpper
  Constant27 : Constant  Value=p.Speed_OutLower
  Constant28 : Constant  Value=p.Speed_IntegUpper
  Constant29 : Constant  Value=p.Speed_IntegLower
  Delay10 : Delay  DelayLength=1  SampleTime=p.SpeedTs
  Gain : Gain  Gain=60/(2*pi)
  Gain6 : Gain  Gain=1/6
  Rate Limiter : RateLimiter  RisingSlewLimit=p.SpeedRef_SlewUp_RPMps  FallingSlewLimit=-p.SpeedRef_SlewDown_RPMps  SampleTimeMode=inherited
  Scope : Scope
      settings: ActiveDisplayYMinimum=-1  ActiveDisplayYMaximum=1  DataLoggingVariableName=ScopeData34
  Scope1 : Scope
      settings: ActiveDisplayYMinimum=-1  ActiveDisplayYMaximum=1  DataLoggingVariableName=ScopeData36
  Speed controller : MATLAB Function  TreatAsAtomicUnit=on
  "Startup_Iq_A " : Constant  Value=p.Startup_Iq_A
  Sum2 : Sum  Inputs=|+-
  Switch : Switch  Criteria=u2 ~= 0  SaturateOnIntegerOverflow=off  InputSameDT=off
  Switch1 : Switch  Criteria=u2 ~= 0  SaturateOnIntegerOverflow=off  InputSameDT=off
  To Workspace : ToWorkspace  Commented=on  VariableName=speederror  SaveFormat=Timeseries  SampleTime=-1
  p.CurrentConvFactor : Gain  Gain=p.CurrentConvFactor
  p.CurrentConvFactorInv : Gain  Gain=p.CurrentConvFactorInv
  p.SpeedUnitsPerRadS : Gain  Gain=p.SpeedUnitsPerRadS
  p.Speed_KiDiv : Gain  Gain=p.Speed_KiDiv
  Iq_raw : Outport
  wires:
  Constant25/1 -> Speed controller/6(KiDiv)
  Switch/1 -> Delay10/1
  Delay10/1 -> Speed controller/2(IqIntegral_prev)
  Constant24/1 -> Speed controller/5(KpDiv)
  Constant27/1 -> Speed controller/8(OutLower)
  Constant29/1 -> Speed controller/10(IntegLower)
  Constant26/1 -> Speed controller/7(OutUpper)
  Speed controller/1(Iq_raw) -> p.CurrentConvFactorInv/1
  omega_mech/1 -> Gain/1, p.SpeedUnitsPerRadS/1  "we"
  Constant28/1 -> Speed controller/9(IntegUpper)
  Constant23/1 -> Speed controller/4(Ki)
  Constant22/1 -> Speed controller/3(Kp)
  p.SpeedUnitsPerRadS/1 -> Sum2/2
  Sum2/1 -> To Workspace/1, Scope/1, Speed controller/1(error)
  reference input in RPM/1 -> Switch1/1
  p.CurrentConvFactorInv/1 -> Scope1/1, Iq_raw/1
  Gain6/1 -> Sum2/1
  Speed controller/2(IqIntegral_next) -> Switch/1
  "Startup_Iq_A "/1 -> p.CurrentConvFactor/1
  p.CurrentConvFactor/1 -> p.Speed_KiDiv/1
  p.Speed_KiDiv/1 -> Switch/3
  phaseNum/1 -> [phaseNum]
  Compare To Constant/1 -> Switch/2
  [phaseNum] -> Compare To Constant/1
  [phaseNum] -> Compare To Constant1/1
  Compare To Constant1/1 -> Switch1/2
  Gain/1 -> Switch1/3
  Switch1/1 -> Rate Limiter/1
  Rate Limiter/1 -> Gain6/1

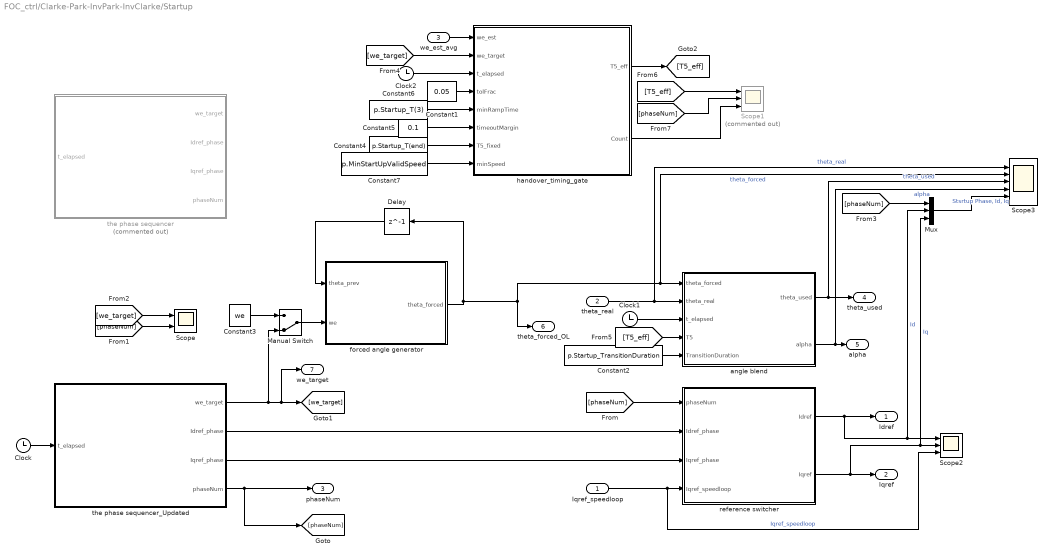
== system FOC_ctrl/Clarke-Park-InvPark-InvClarke/Startup ==
  "Iqref_speedloop " : Inport
  "theta_real " : Inport  Port=2
  we_est_avg : Inport  Port=3
  " reference switcher" : MATLAB Function  TreatAsAtomicUnit=on
  Clock : Clock
  Clock1 : Clock
  Clock2 : Clock
  Constant1 : Constant  Value=0.05
  Constant2 : Constant  Value=p.Startup_TransitionDuration
  Constant3 : Constant  Value=we
  Constant4 : Constant  Value=p.Startup_T(end)
  Constant5 : Constant  Value=0.1
  Constant6 : Constant  Value=p.Startup_T(3)
  Constant7 : Constant  Value=p.MinStartUpValidSpeed
  Delay : Delay  DelayLength=1  SampleTime=p.Ts
  Manual Switch : ManualSwitch  CurrentSetting=0
  Mux : Mux  Inputs=3
  Scope : Scope  NumInputPorts=2
      settings: ActiveDisplayYMinimum=-99.352867669777183  ActiveDisplayYMaximum=894.17580902799489  DataLoggingVariableName=ScopeData32
  Scope1 : Scope  Commented=on  NumInputPorts=3
      settings: ActiveDisplayYMinimum=0.619736375  ActiveDisplayYMaximum=0.62336262500000006  DataLoggingVariableName=ScopeData26
  Scope2 : Scope  NumInputPorts=3
      settings: ActiveDisplayYMinimum=-1.2499999999999998  ActiveDisplayYMaximum=11.25  DataLoggingVariableName=ScopeData33
  Scope3 : Scope  NumInputPorts=5
      settings: ActiveDisplayYMinimum=-3.9267263512221913  ActiveDisplayYMaximum=3.9260768541659612  DataLoggingVariableName=ScopeData23
  angle blend : MATLAB Function  TreatAsAtomicUnit=on
  forced angle generator : MATLAB Function  TreatAsAtomicUnit=on
  handover_timing_gate : MATLAB Function  TreatAsAtomicUnit=on
  the phase sequencer : MATLAB Function  Commented=on  TreatAsAtomicUnit=on
  the phase sequencer_Updated : MATLAB Function  TreatAsAtomicUnit=on
  Idref : Outport
  Iqref : Outport  Port=2
  phaseNum : Outport  Port=3
  theta_used : Outport  Port=4
  alpha : Outport  Port=5
  theta_forced_OL : Outport  Port=6
  we_target : Outport  Port=7
  wires:
  Clock/1 -> the phase sequencer_Updated/1(t_elapsed)
  the phase sequencer_Updated/2(Idref_phase) -> " reference switcher"/2(Idref_phase)
  the phase sequencer_Updated/3(Iqref_phase) -> " reference switcher"/3(Iqref_phase)
  the phase sequencer_Updated/4(phaseNum) -> phaseNum/1, [phaseNum]
  forced angle generator/1(theta_forced) -> Delay/1, Scope3/2, angle blend/1(theta_forced), theta_forced_OL/1  "theta_forced"
  Delay/1 -> forced angle generator/1(theta_prev)
  " reference switcher"/2(Iqref) -> Mux/3, Scope2/2, Iqref/1  "Iq"
  " reference switcher"/1(Idref) -> Mux/2, Scope2/1, Idref/1  "Id"
  Clock1/1 -> angle blend/3(t_elapsed)
  [T5_eff] -> angle blend/4(T5)
  Constant2/1 -> angle blend/5(TransitionDuration)
  angle blend/1(theta_used) -> Scope3/3, theta_used/1  "theta_used"
  angle blend/2(alpha) -> Scope3/4, alpha/1  "alpha"
  [phaseNum] -> " reference switcher"/1(phaseNum)
  [phaseNum] -> Scope/2
  "Iqref_speedloop "/1 -> Scope2/3, " reference switcher"/4(Iqref_speedloop)  "Iqref_speedloop"
  "theta_real "/1 -> Scope3/1, angle blend/2(theta_real)  "theta_real"
  Constant3/1 -> Manual Switch/1
  Manual Switch/1 -> forced angle generator/2(we)
  the phase sequencer_Updated/1(we_target) -> we_target/1, [we_target], Manual Switch/2
  [we_target] -> Scope/1
  Mux/1 -> Scope3/5  "Stsrtup Phase, Id, Iq"
  [phaseNum] -> Mux/1
  we_est_avg/1 -> handover_timing_gate/1(we_est)
  [we_target] -> handover_timing_gate/2(we_target)
  Clock2/1 -> handover_timing_gate/3(t_elapsed)
  Constant4/1 -> handover_timing_gate/7(T5_fixed)
  Constant5/1 -> handover_timing_gate/6(timeoutMargin)
  Constant6/1 -> handover_timing_gate/5(minRampTime)
  handover_timing_gate/1(T5_eff) -> [T5_eff]
  [T5_eff] -> Scope1/1
  [phaseNum] -> Scope1/2
  Constant1/1 -> handover_timing_gate/4(tolFrac)
  Constant7/1 -> handover_timing_gate/8(minSpeed)
  handover_timing_gate/2(Count) -> Scope1/3

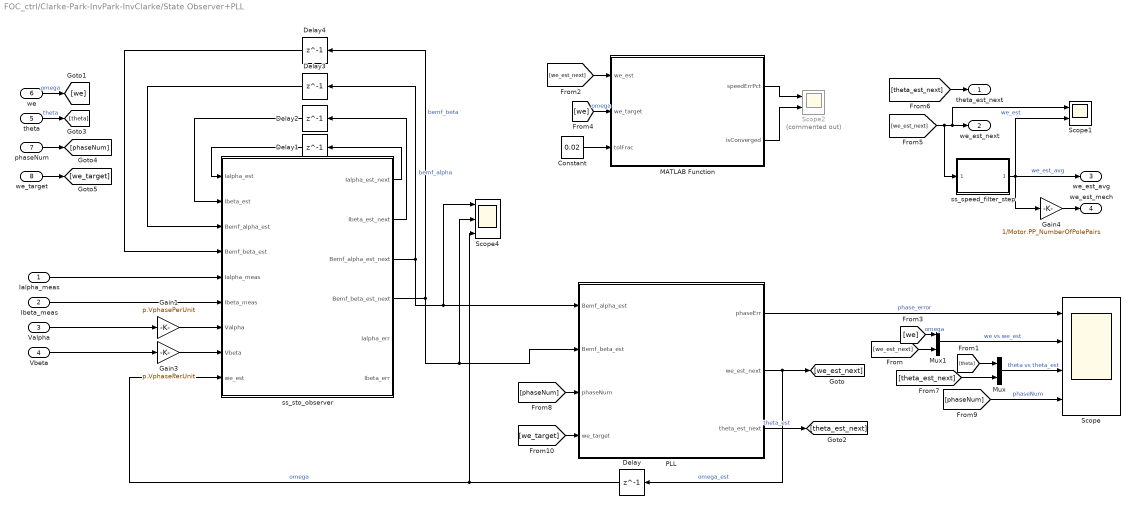
== system FOC_ctrl/Clarke-Park-InvPark-InvClarke/State Observer+PLL ==
  Ialpha_meas : Inport
  Ibeta_meas : Inport  Port=2
  Valpha : Inport  Port=3
  Vbeta : Inport  Port=4
  theta : Inport  Port=5
  we : Inport  Port=6
  phaseNum : Inport  Port=7
  we_target : Inport  Port=8
  Constant : Constant  Value=0.02
  Delay{,1..4} (5 alike) : Delay  DelayLength=1  SampleTime=p.Ts
  Gain1 : Gain  Gain=p.VphasePerUnit
  Gain3 : Gain  Gain=p.VphasePerUnit
  Gain4 : Gain  Gain=1/Motor.PP_NumberOfPolePairs
  MATLAB Function : MATLAB Function  TreatAsAtomicUnit=on
  Mux : Mux  Inputs=2
  Mux1 : Mux  Inputs=2
  PLL : Subsystem
  Scope : Scope  NumInputPorts=4
      settings: ActiveDisplayYMinimum=-530.68047991486117  ActiveDisplayYMaximum=1413.3873683092527  DataLoggingVariableName=ScopeData22
  Scope1 : Scope  NumInputPorts=2
      settings: ActiveDisplayYMinimum=-1  ActiveDisplayYMaximum=1  DataLoggingVariableName=ScopeData37
  Scope2 : Scope  Commented=on  NumInputPorts=2
      settings: ActiveDisplayYMinimum=-124.86192949822214  ActiveDisplayYMaximum=1123.8735477220248  DataLoggingVariableName=ScopeData31
  Scope4 : Scope  NumInputPorts=3
      settings: ActiveDisplayYMinimum=-8.6149655089635218  ActiveDisplayYMaximum=8.3845226438040683  DataLoggingVariableName=ScopeData38
  ss_speed_filter_step : MATLAB Function  TreatAsAtomicUnit=on
  ss_sto_observer : MATLAB Function  TreatAsAtomicUnit=on
  theta_est_next : Outport
  we_est_next : Outport  Port=2
  we_est_avg : Outport  Port=3
  we_est_mech : Outport  Port=4
  wires:
  Ialpha_meas/1 -> ss_sto_observer/5(Ialpha_meas)
  Ibeta_meas/1 -> ss_sto_observer/6(Ibeta_meas)
  PLL/2(we_est_next) -> [we_est_next], Delay/1  "omega_est"
  Delay/1 -> Scope4/3, ss_sto_observer/9(we_est)  "omega"
  ss_sto_observer/3(Bemf_alpha_est_next) -> Scope4/1, PLL/1(Bemf_alpha_est), Delay3/1  "bemf_alpha"
  ss_sto_observer/4(Bemf_beta_est_next) -> Scope4/2, PLL/2(Bemf_beta_est), Delay4/1  "bemf_beta"
  ss_sto_observer/1(Ialpha_est_next) -> Delay1/1
  Delay1/1 -> ss_sto_observer/1(Ialpha_est)
  ss_sto_observer/2(Ibeta_est_next) -> Delay2/1
  Delay2/1 -> ss_sto_observer/2(Ibeta_est)
  Delay3/1 -> ss_sto_observer/3(Bemf_alpha_est)
  Delay4/1 -> ss_sto_observer/4(Bemf_beta_est)
  PLL/3(theta_est_next) -> [theta_est_next]  "theta_est"
  PLL/1(phaseErr) -> Scope/1  "phase_error"
  theta/1 -> [theta]  "theta"
  Mux/1 -> Scope/3  "theta vs theta_est"
  [we] -> Mux1/1  "omega"
  Mux1/1 -> Scope/2  "we vs we_est"
  Valpha/1 -> Gain1/1
  Gain1/1 -> ss_sto_observer/7(Valpha)
  Vbeta/1 -> Gain3/1
  Gain3/1 -> ss_sto_observer/8(Vbeta)
  [we_est_next] -> Mux1/2
  [we_est_next] -> MATLAB Function/1(we_est)
  we/1 -> [we]  "omega"
  [we] -> MATLAB Function/2(we_target)  "omega"
  Constant/1 -> MATLAB Function/3(tolFrac)
  MATLAB Function/1(speedErrPct) -> Scope2/1
  MATLAB Function/2(isConverged) -> Scope2/2
  [theta_est_next] -> theta_est_next/1
  [theta_est_next] -> Mux/2
  [theta] -> Mux/1
  phaseNum/1 -> [phaseNum]
  [phaseNum] -> PLL/3(phaseNum)
  [phaseNum] -> Scope/4  "phaseNum"
  [we_target] -> PLL/4(we_target)
  we_target/1 -> [we_target]
  [we_est_next] -> ss_speed_filter_step/1(we_est), Scope1/1, we_est_next/1  "we_est"
  ss_speed_filter_step/1(we_avg) -> Gain4/1, we_est_avg/1, Scope1/2  "we_est_avg"
  Gain4/1 -> we_est_mech/1

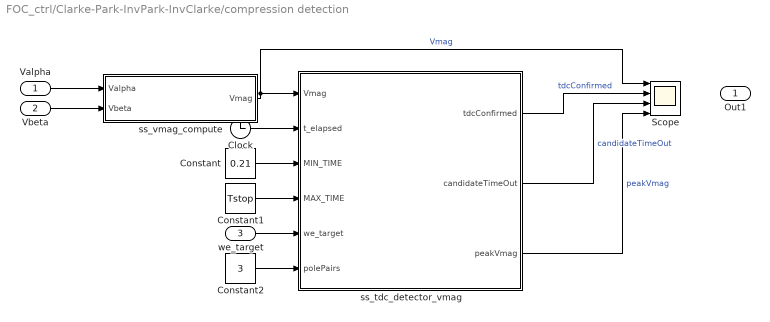
== system FOC_ctrl/Clarke-Park-InvPark-InvClarke/compression detection ==
  Valpha : Inport
  Vbeta : Inport  Port=2
  we_target : Inport  Port=3
  Clock : Clock
  Constant : Constant  Value=0.21
  Constant1 : Constant  Value=Tstop
  Constant2 : Constant  Value=3
  Scope : Scope  NumInputPorts=4
      settings: ActiveDisplayYMinimum=0.059733582495011789  ActiveDisplayYMaximum=1.5647113379151045  DataLoggingVariableName=ScopeData42
  ss_tdc_detector_vmag : MATLAB Function  TreatAsAtomicUnit=on
  ss_vmag_compute : MATLAB Function  TreatAsAtomicUnit=on
  Out1 : Outport
  wires:
  ss_vmag_compute/1(Vmag) -> ss_tdc_detector_vmag/1(Vmag), Scope/1  "Vmag"
  Valpha/1 -> ss_vmag_compute/1(Valpha)
  Vbeta/1 -> ss_vmag_compute/2(Vbeta)
  Constant/1 -> ss_tdc_detector_vmag/3(MIN_TIME)
  Constant1/1 -> ss_tdc_detector_vmag/4(MAX_TIME)
  Clock/1 -> ss_tdc_detector_vmag/2(t_elapsed)
  ss_tdc_detector_vmag/1(tdcConfirmed) -> Scope/2  "tdcConfirmed"
  ss_tdc_detector_vmag/2(candidateTimeOut) -> Scope/3  "candidateTimeOut"
  ss_tdc_detector_vmag/3(peakVmag) -> Scope/4  "peakVmag"
  Constant2/1 -> ss_tdc_detector_vmag/6(polePairs)
  we_target/1 -> ss_tdc_detector_vmag/5(we_target)

== system FOC_ctrl/Cogging Torque/Variant Subsystem ==
  note: 1) Add Subsystem or Model blocks as valid variant choices.
      | 2) You cannot connect blocks at this level. At simulation, connectivity is automatically
      | determined, based on the active variant and port name matching.
  theta : Inport
  BD Nano : Subsystem  VariantControl=Option.Product==1
  BD Nano Lite : Subsystem  VariantControl=Option.Product==4
  Tcog : Outport
